simulink model "w4_001_lab_11march"  (R2023b)
settings: Solver=VariableStepAuto  StartTime=0.0  StopTime=15  RelTol=1e-3
settings Model: Creator=Aksel Cavak  LastModifiedBy=Aksel Cavak

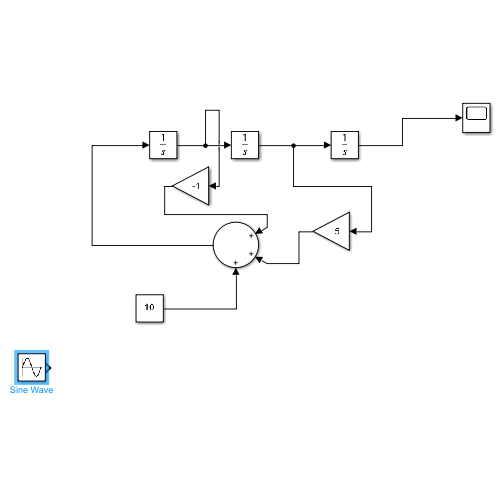
[thumbnail: Simulink's stored preview of the top-level diagram]
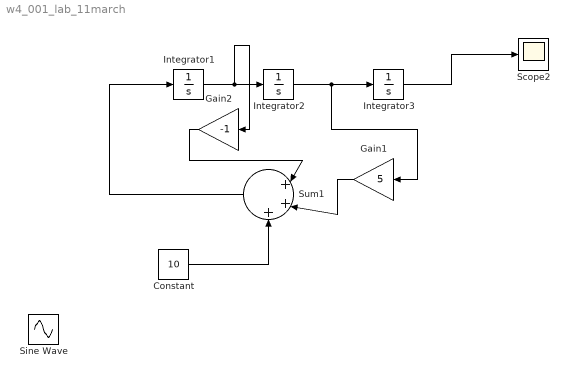
== system w4_001_lab_11march ==
  Constant : Constant  Value=10
  Gain1 : Gain  Gain=5
  Gain2 : Gain  Gain=-1
  Integrator1 : Integrator
  Integrator2 : Integrator
  Integrator3 : Integrator
  Scope2 : Scope
  Sine Wave : Sin  Amplitude=2  Frequency=0.5  SampleTime=0
  Sum1 : Sum  Inputs=|+++
  wires:
  Integrator2/1 -> Gain1/1, Integrator3/1
  Integrator3/1 -> Scope2/1
  Gain1/1 -> Sum1/2
  Sum1/1 -> Integrator1/1
  Integrator1/1 -> Gain2/1, Integrator2/1
  Constant/1 -> Sum1/3
  Gain2/1 -> Sum1/1
